simulink model "llc"  (R2020a)
settings: Solver=VariableStepAuto  StartTime=0.0  StopTime=0.1  RelTol=1e-3
values from neighbouring files (symbols this model uses):
  LLC_PLANT_F_RES = 87.5e3    (= 87500)    [llc_init_cfg.m]
  LLC_PLANT_K = 0.000952281115447026    (= 0.000952281115447)    [llc_init_cfg.m]
  LLC_PLANT_Q = 0.5    [llc_init_cfg.m]
libraries: powerlib x17, commsynccomp2 x2, simulink x2
settings Model: Creator=huyan  LastModifiedBy=huyan

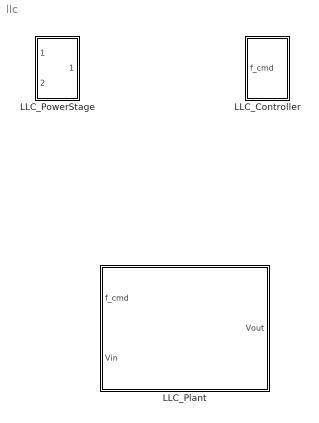
== system llc ==
  LLC_Controller : Subsystem
  LLC_Plant : Subsystem
  LLC_PowerStage : Subsystem

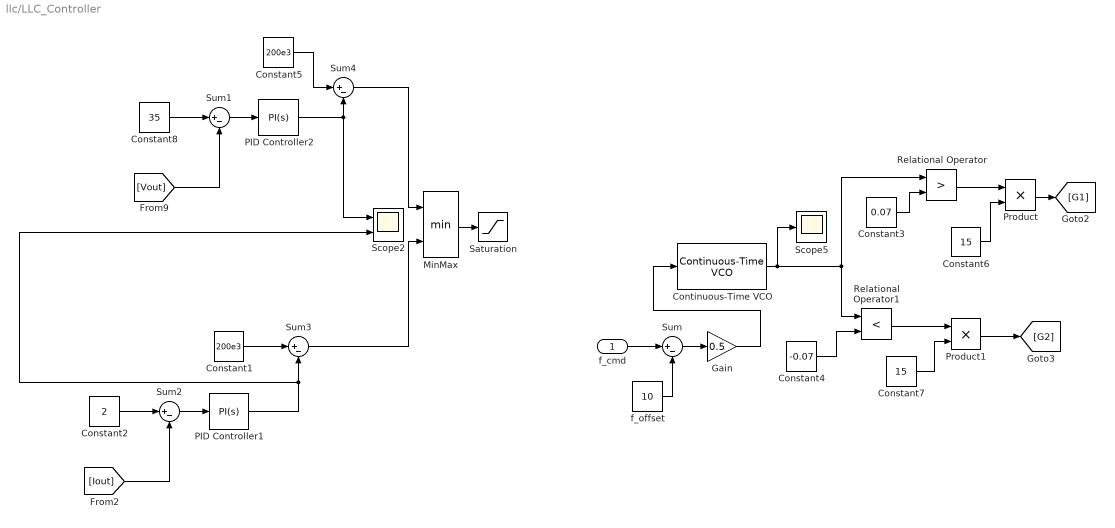
== system llc/LLC_Controller ==
  f_cmd : Inport
  Constant1 : Constant  Value=200e3
  Constant2 : Constant  Value=2
  Constant3 : Constant  Value=0.07
  Constant4 : Constant  Value=-0.07
  Constant5 : Constant  Value=200e3
  Constant6 : Constant  Value=15
  Constant7 : Constant  Value=15
  Constant8 : Constant  Value=35
  Continuous-Time VCO : commsynccomp2/Continuous-Time VCO  Ac=1  Fc=10  Kc=2  Ph=0
      settings: SourceProductBaseCode=CM
  Gain : Gain  Gain=0.5
  MinMax : MinMax  Inputs=2
  PID Controller1 : simulink/Continuous/PID Controller  Controller=PI  Form=Parallel  TimeDomain=Continuous-time  UseExternalTs=off  SampleTime=-1  IntegratorMethod=Forward Euler  FilterMethod=Forward Euler  ControllerParametersSource=internal  P=1000  I=1000000  D=0  UseFilter=on  N=100  TunerSelectOption=Transfer Function Based (PID Tuner App)  InitialConditionSource=internal  InitialConditionForIntegrator=0  InitialConditionForFilter=0  DifferentiatorICPrevScaledInput=0  ExternalReset=none  TrackingMode=off  Kt=1  LimitOutput=off  UpperSaturationLimit=inf  LowerSaturationLimit=-inf  LinearizeAsGain=on  AntiWindupMode=none  Kb=1  POutMin=[]  POutMax=[]  IOutMin=[]  IOutMax=[]  DOutMin=[]  DOutMax=[]  NOutMin=[]  NOutMax=[]  SumOutMin=[]  SumOutMax=[]  SaturationOutMin=[]  SaturationOutMax=[]  PParamMin=[]  PParamMax=[]  IParamMin=[]  IParamMax=[]  DParamMin=[]  DParamMax=[]  NParamMin=[]  NParamMax=[]  KbParamMin=[]  KbParamMax=[]  KtParamMin=[]  KtParamMax=[]  KbOutMin=[]  KbOutMax=[]  KtOutMin=[]  KtOutMax=[]  IntegratorOutMin=[]  IntegratorOutMax=[]  FilterOutMin=[]  FilterOutMax=[]  SumI1OutMin=[]  SumI1OutMax=[]  SumI2OutMin=[]  SumI2OutMax=[]  SumI3OutMin=[]  SumI3OutMax=[]  SumI4OutMin=[]  SumI4OutMax=[]  SumDOutMin=[]  SumDOutMax=[]  DifferentiatorOutMin=[]  DifferentiatorOutMax=[]  FilterDiffOutCoefMin=[]  FilterDiffOutCoefMax=[]  ReciprocalOutMin=[]  ReciprocalOutMax=[]  SumDenOutMin=[]  SumDenOutMax=[]  SumNumOutMin=[]  SumNumOutMax=[]  DivideOutMin=[]  DivideOutMax=[]  UdiffTsProdOutMin=[]  UdiffTsProdOutMax=[]  NTsProdOutMin=[]  NTsProdOutMax=[]  UintegralTsProdOutMin=[]  UintegralTsProdOutMax=[]  UngainTsProdOutMin=[]  UngainTsProdOutMax=[]  IntegratorContinuousStateAttributes=''  IntegratorStateMustResolveToSignalObject=off  IntegratorRTWStateStorageClass=Auto  FilterContinuousStateAttributes=''  FilterStateMustResolveToSignalObject=off  FilterRTWStateStorageClass=Auto  ParallelPVariant=InternalParameters  IdealPVariant=Disabled  IVariant=InternalParameters  DVariant=Disabled  IntegratorVariant=Continuous  SatVariant=Disabled  AWVariant=Passthrough  PCopyVariant=Disabled  TRVariant=Disabled  FdbkBlocksVariant=Forward  IdealPFdbkVariant=Disabled  SatFdbkVariant=Disabled  DerivativeFilterVariant=Disabled  NVariant=Disabled  NCopyVariant=Disabled_SignalSpec  FilterICVariant=Disabled  IntegratorICVariant=InternalICs  ExternalResetVariant=Disabled  TRSumVariant=Passthrough  SumFdbkVariant=Disabled  SumVariant=Sum_PI  TsampFilterVariant=InternalTs  TsampNgainVariant=Passthrough  TsampIntegralVariant=Passthrough
  PID Controller2 : simulink/Continuous/PID Controller  Controller=PI  Form=Parallel  TimeDomain=Continuous-time  UseExternalTs=off  SampleTime=-1  IntegratorMethod=Forward Euler  FilterMethod=Forward Euler  ControllerParametersSource=internal  P=1000  I=1000000  D=0  UseFilter=on  N=100  TunerSelectOption=Transfer Function Based (PID Tuner App)  InitialConditionSource=internal  InitialConditionForIntegrator=0  InitialConditionForFilter=0  DifferentiatorICPrevScaledInput=0  ExternalReset=none  TrackingMode=off  Kt=1  LimitOutput=off  UpperSaturationLimit=inf  LowerSaturationLimit=-inf  LinearizeAsGain=on  AntiWindupMode=none  Kb=1  POutMin=[]  POutMax=[]  IOutMin=[]  IOutMax=[]  DOutMin=[]  DOutMax=[]  NOutMin=[]  NOutMax=[]  SumOutMin=[]  SumOutMax=[]  SaturationOutMin=[]  SaturationOutMax=[]  PParamMin=[]  PParamMax=[]  IParamMin=[]  IParamMax=[]  DParamMin=[]  DParamMax=[]  NParamMin=[]  NParamMax=[]  KbParamMin=[]  KbParamMax=[]  KtParamMin=[]  KtParamMax=[]  KbOutMin=[]  KbOutMax=[]  KtOutMin=[]  KtOutMax=[]  IntegratorOutMin=[]  IntegratorOutMax=[]  FilterOutMin=[]  FilterOutMax=[]  SumI1OutMin=[]  SumI1OutMax=[]  SumI2OutMin=[]  SumI2OutMax=[]  SumI3OutMin=[]  SumI3OutMax=[]  SumI4OutMin=[]  SumI4OutMax=[]  SumDOutMin=[]  SumDOutMax=[]  DifferentiatorOutMin=[]  DifferentiatorOutMax=[]  FilterDiffOutCoefMin=[]  FilterDiffOutCoefMax=[]  ReciprocalOutMin=[]  ReciprocalOutMax=[]  SumDenOutMin=[]  SumDenOutMax=[]  SumNumOutMin=[]  SumNumOutMax=[]  DivideOutMin=[]  DivideOutMax=[]  UdiffTsProdOutMin=[]  UdiffTsProdOutMax=[]  NTsProdOutMin=[]  NTsProdOutMax=[]  UintegralTsProdOutMin=[]  UintegralTsProdOutMax=[]  UngainTsProdOutMin=[]  UngainTsProdOutMax=[]  IntegratorContinuousStateAttributes=''  IntegratorStateMustResolveToSignalObject=off  IntegratorRTWStateStorageClass=Auto  FilterContinuousStateAttributes=''  FilterStateMustResolveToSignalObject=off  FilterRTWStateStorageClass=Auto  ParallelPVariant=InternalParameters  IdealPVariant=Disabled  IVariant=InternalParameters  DVariant=Disabled  IntegratorVariant=Continuous  SatVariant=Disabled  AWVariant=Passthrough  PCopyVariant=Disabled  TRVariant=Disabled  FdbkBlocksVariant=Forward  IdealPFdbkVariant=Disabled  SatFdbkVariant=Disabled  DerivativeFilterVariant=Disabled  NVariant=Disabled  NCopyVariant=Disabled_SignalSpec  FilterICVariant=Disabled  IntegratorICVariant=InternalICs  ExternalResetVariant=Disabled  TRSumVariant=Passthrough  SumFdbkVariant=Disabled  SumVariant=Sum_PI  TsampFilterVariant=InternalTs  TsampNgainVariant=Passthrough  TsampIntegralVariant=Passthrough
  Product : Product
  Product1 : Product
  Relational Operator : RelationalOperator  Operator=>  OutDataTypeStr=boolean  RndMeth=Simplest
  Relational Operator1 : RelationalOperator  Operator=<  OutDataTypeStr=boolean  RndMeth=Simplest
  Saturation : Saturate  UpperLimit=150e3  LowerLimit=35e3
  Scope2 : Scope  NumInputPorts=2
  Scope5 : Scope
  Sum{,1..4} (5 alike) : Sum  Inputs=|+-
  f_offset : Constant  Value=10
  wires:
  PID Controller2/1 -> Scope2/1, Sum4/2
  Constant3/1 -> Relational Operator/2
  Continuous-Time VCO/1 -> Scope5/1, Relational Operator/1, Relational Operator1/1
  [Iout] -> Sum2/2
  MinMax/1 -> Saturation/1
  Constant6/1 -> Product/2
  Sum3/1 -> MinMax/2
  Constant5/1 -> Sum4/1
  Sum1/1 -> PID Controller2/1
  Relational Operator/1 -> Product/1
  Sum2/1 -> PID Controller1/1
  Constant1/1 -> Sum3/1
  Sum4/1 -> MinMax/1
  Constant8/1 -> Sum1/1
  PID Controller1/1 -> Scope2/2, Sum3/2
  [Vout] -> Sum1/2
  Product/1 -> [G1]
  Relational Operator1/1 -> Product1/1
  Constant7/1 -> Product1/2
  Constant4/1 -> Relational Operator1/2
  Constant2/1 -> Sum2/1
  Product1/1 -> [G2]
  f_cmd/1 -> Sum/1
  f_offset/1 -> Sum/2
  Sum/1 -> Gain/1
  Gain/1 -> Continuous-Time VCO/1

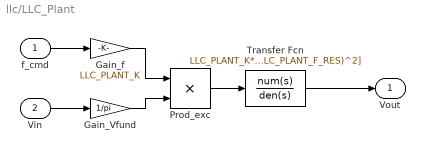
== system llc/LLC_Plant ==
  f_cmd : Inport
  Vin : Inport  Port=2
  Gain_Vfund : Gain  Gain=1/pi
  Gain_f : Gain  Gain=LLC_PLANT_K
  Prod_exc : Product  Inputs=**
  Transfer Fcn : TransferFcn  Numerator=LLC_PLANT_K*(2*pi*LLC_PLANT_F_RES)^2  Denominator=[1, 2*LLC_PLANT_Q*(2*pi*LLC_PLANT_F_RES), (2*pi*LLC_PLANT_F_RES)^2]
  Vout : Outport
  wires:
  f_cmd/1 -> Gain_f/1
  Vin/1 -> Gain_Vfund/1
  Gain_f/1 -> Prod_exc/1
  Gain_Vfund/1 -> Prod_exc/2
  Prod_exc/1 -> Transfer Fcn/1
  Transfer Fcn/1 -> Vout/1

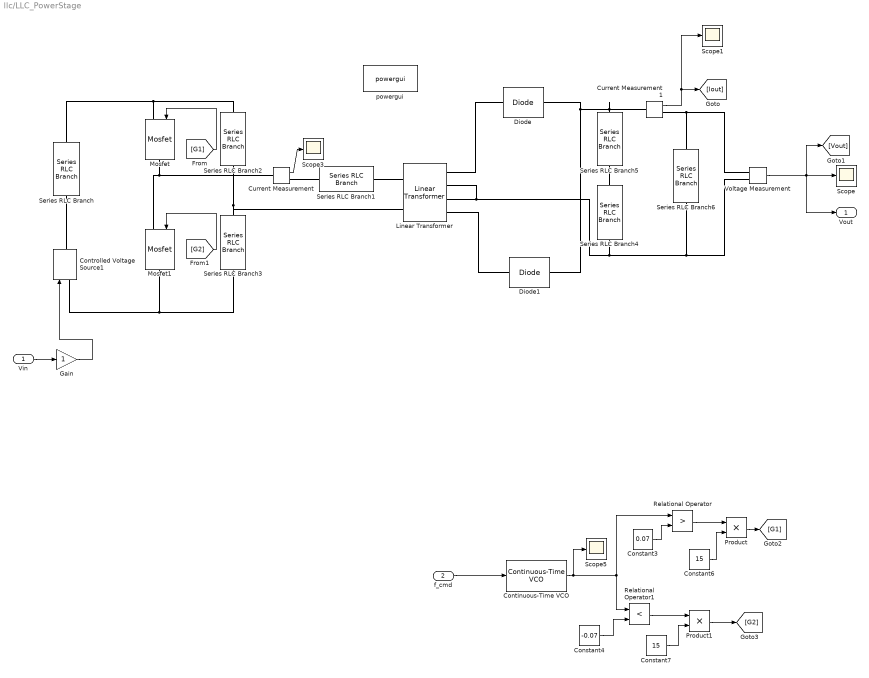
== system llc/LLC_PowerStage ==
  Vin : Inport
  f_cmd : Inport  Port=2
  Constant3 : Constant  Value=0.07
  Constant4 : Constant  Value=-0.07
  Constant6 : Constant  Value=15
  Constant7 : Constant  Value=15
  Continuous-Time VCO : commsynccomp2/Continuous-Time VCO  Ac=1  Fc=0  Kc=1  Ph=0
      settings: SourceProductBaseCode=CM
  Controlled Voltage Source1 : powerlib/Electrical Sources/Controlled Voltage Source  Initialize=on  Source_Type=AC  Amplitude=0  Phase=0  Frequency=0  Measurements=None
  Current Measurement : powerlib/Measurements/Current Measurement  PhasorSimulation=off  OutputType=Complex  PSBequivalent=0
  Current Measurement1 : powerlib/Measurements/Current Measurement  PhasorSimulation=off  OutputType=Complex  PSBequivalent=0
  Diode : powerlib/Power Electronics/Diode  Ron=0.001  Lon=0  Vf=1.5  IC=0  UseSnubber=0  Rs=0.8  Cs=1e-9  Measurements=off
  Diode1 : powerlib/Power Electronics/Diode  Ron=0.001  Lon=0  Vf=1.5  IC=0  UseSnubber=0  Rs=0.8  Cs=1e-9  Measurements=off
  Gain : Gain
  Linear Transformer : powerlib/Elements/Linear Transformer  UNITS=SI  NominalPower=[ 3000 100000 ]  winding1=[300 0 0]  winding2=[80 0 0]  ThreeWindings=on  winding3=[80 0 0]  RmLm=[2.888e+08 0.00077]  Measurements=None  DataType=on
  Mosfet : powerlib/Power Electronics/Mosfet  Ron=0.1  Lon=0  Rd=0.01  Vfd=0  IC=0  Rs=1e5  Cs=inf  Measurements=off
  Mosfet1 : powerlib/Power Electronics/Mosfet  Ron=0.1  Lon=0  Rd=0.01  Vfd=0  IC=0  Rs=1e5  Cs=inf  Measurements=off
  Product : Product
  Product1 : Product
  Relational Operator : RelationalOperator  Operator=>  OutDataTypeStr=boolean  RndMeth=Simplest
  Relational Operator1 : RelationalOperator  Operator=<  OutDataTypeStr=boolean  RndMeth=Simplest
  Scope{,1,3,5} (4 alike) : Scope
  Series RLC Branch : powerlib/Elements/Series RLC Branch  LConnTagsString=__new0  RConnTagsString=__new0  BranchType=R  Resistance=1E-3  Inductance=1e-3  SetiL0=off  InitialCurrent=0  Capacitance=1e-6  Setx0=off  InitialVoltage=0  Measurements=None
  Series RLC Branch1 : powerlib/Elements/Series RLC Branch  LConnTagsString=__new0  RConnTagsString=__new0  BranchType=L  Resistance=1E-3  Inductance=23e-6  SetiL0=off  InitialCurrent=0  Capacitance=1e-6  Setx0=off  InitialVoltage=0  Measurements=None
  Series RLC Branch2 : powerlib/Elements/Series RLC Branch  LConnTagsString=__new0  RConnTagsString=__new0  BranchType=C  Resistance=1E-3  Inductance=23e-3  SetiL0=off  InitialCurrent=0  Capacitance=66e-9  Setx0=off  InitialVoltage=0  Measurements=None
  Series RLC Branch3 : powerlib/Elements/Series RLC Branch  LConnTagsString=__new0  RConnTagsString=__new0  BranchType=C  Resistance=1E-3  Inductance=23e-3  SetiL0=off  InitialCurrent=0  Capacitance=66e-9  Setx0=off  InitialVoltage=0  Measurements=None
  Series RLC Branch4 : powerlib/Elements/Series RLC Branch  LConnTagsString=__new0  RConnTagsString=__new0  BranchType=C  Resistance=1E-3  Inductance=23e-3  SetiL0=off  InitialCurrent=0  Capacitance=12000e-6  Setx0=off  InitialVoltage=0  Measurements=None
  Series RLC Branch5 : powerlib/Elements/Series RLC Branch  LConnTagsString=__new0  RConnTagsString=__new0  BranchType=R  Resistance=0.025  Inductance=1e-3  SetiL0=off  InitialCurrent=0  Capacitance=1e-6  Setx0=off  InitialVoltage=0  Measurements=None
  Series RLC Branch6 : powerlib/Elements/Series RLC Branch  LConnTagsString=__new0  RConnTagsString=__new0  BranchType=R  Resistance=1.36875  Inductance=1e-3  SetiL0=off  InitialCurrent=0  Capacitance=1e-6  Setx0=off  InitialVoltage=0  Measurements=None
  Voltage Measurement : powerlib/Measurements/Voltage Measurement  PhasorSimulation=off  OutputType=Complex  PSBequivalent=0
  powergui : powerlib/powergui  Priority=1  SimulationMode=Discrete  SampleTime=1e-7  frequency=60  Iterations=50  frequencyindice=0  Pbase=100e6  ErrMax=1e-4  UnitsV=kV  UnitsW=MW  buscounter=0  FunctionMessages=off  echomessages=off  EnableUseOfTLC=off  CurrentSourceSwitches=off  DisableSnubberDevices=off  DisableRonSwitches=off  DisableVfSwitches=off  DisplayEquations=off  AutomaticDiscreteSolvers=off  SolverType=Tustin/Backward Euler (TBE)  Interpol=off  ExternalGateDelay=off  methode=off  Ts=100  x0status=blocks  SPID=on  SwTol=0  HookPort=off  NonlinearTolerance=1e-4  nMaxIteration=100  ContinueOnMaxIteration=off  RestoreLinks=warning  ResistiveCurrentMeasurement=off  Frange=[0:2:500]  Ylog=off  Xlog=on  ShowGrid=off  save=off  variable=ZData  structure=0  ZoomFFT=off  StartTime=0.0  cycles=1  DisplayStyle=1  fundamental=60  FreqAxis=off  MaxFrequency=1000  frequencyindicesteady=1  RmsSteady=1  display=off
  Vout : Outport
  wires:
  [G2] -> Mosfet1/1
  Current Measurement1/1 -> Scope1/1, [Iout]
  [G1] -> Mosfet/1
  Current Measurement/1 -> Scope3/1
  Vin/1 -> Gain/1
  Gain/1 -> Controlled Voltage Source1/1
  Voltage Measurement/1 -> Vout/1, Scope/1, [Vout]
  Product1/1 -> [G2]
  Constant4/1 -> Relational Operator1/2
  Product/1 -> [G1]
  Relational Operator1/1 -> Product1/1
  Relational Operator/1 -> Product/1
  Continuous-Time VCO/1 -> Scope5/1, Relational Operator/1, Relational Operator1/1
  Constant3/1 -> Relational Operator/2
  Constant6/1 -> Product/2
  Constant7/1 -> Product1/2
  f_cmd/1 -> Continuous-Time VCO/1
  connections:
  Series RLC Branch/LConn1 -- Mosfet/LConn1 -- Series RLC Branch2/LConn1
  Current Measurement/RConn1 -- Series RLC Branch1/RConn1
  Mosfet/RConn1 -- Mosfet1/LConn1 -- Current Measurement/LConn1
  Controlled Voltage Source1/RConn1 -- Series RLC Branch/RConn1
  Series RLC Branch6/RConn1 -- Voltage Measurement/LConn2 -- Series RLC Branch4/RConn1 -- Linear Transformer/RConn2 -- Linear Transformer/RConn3
  Series RLC Branch3/LConn1 -- Controlled Voltage Source1/LConn1 -- Mosfet1/RConn1
  Diode/RConn1 -- Series RLC Branch5/LConn1 -- Current Measurement1/LConn1 -- Diode1/RConn1
  Series RLC Branch2/RConn1 -- Linear Transformer/LConn2 -- Series RLC Branch3/RConn1
  Linear Transformer/RConn1 -- Diode/LConn1
  Current Measurement1/RConn1 -- Voltage Measurement/LConn1 -- Series RLC Branch6/LConn1
  Series RLC Branch1/LConn1 -- Linear Transformer/LConn1
  Linear Transformer/RConn4 -- Diode1/LConn1
  Series RLC Branch5/RConn1 -- Series RLC Branch4/LConn1
